simulink model "buck_discrete_pi_voltage_loop"  (R2024b)
settings: Solver=ode4  StartTime=0.0  StopTime=0.012  FixedStep=2.5e-7  RelTol=1e-3
undefined symbols (not defined in the file): DiscIntNeverNeededParam
settings Model: Creator=ww  LastModifiedBy=ww

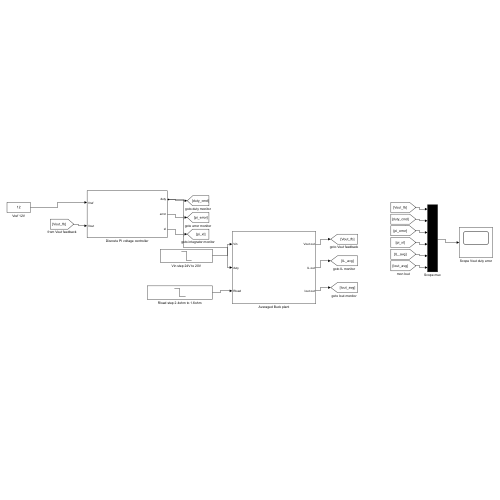
[thumbnail: Simulink's stored preview of the top-level diagram]
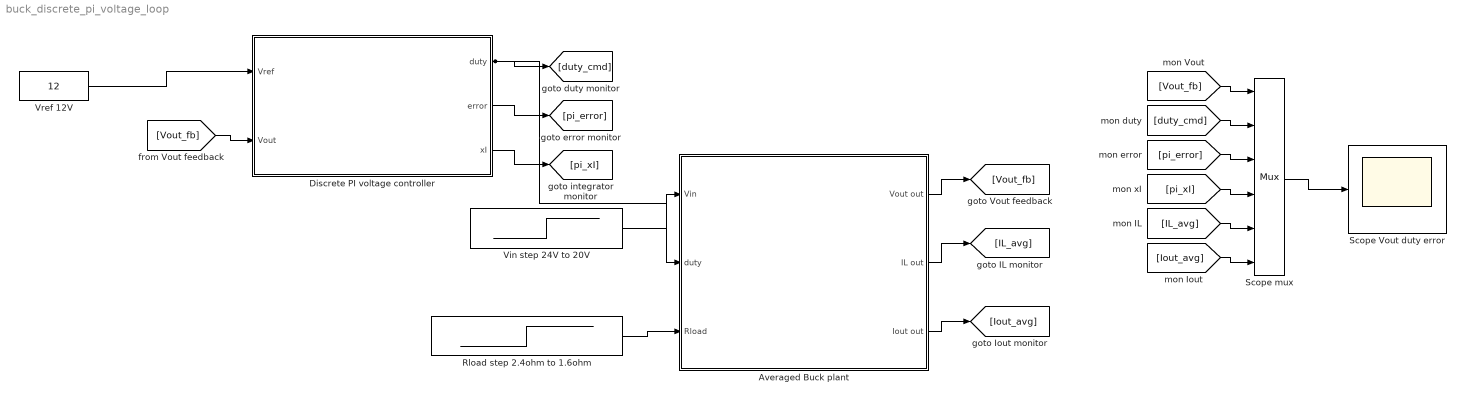
== system buck_discrete_pi_voltage_loop ==
  Averaged Buck plant : Subsystem
  Discrete PI voltage controller : Subsystem
  Rload step 2.4ohm to 1.6ohm : Step  Time=0.007  Before=2.4  After=1.6  SampleTime=0
  Scope Vout duty error : Scope
  Scope mux : Mux  Inputs=6
  Vin step 24V to 20V : Step  Time=0.003  Before=24  After=20  SampleTime=0
  Vref 12V : Constant  Value=12
  wires:
  [Vout_fb] -> Scope mux/1
  [duty_cmd] -> Scope mux/2
  [pi_error] -> Scope mux/3
  [pi_xI] -> Scope mux/4
  [IL_avg] -> Scope mux/5
  [Iout_avg] -> Scope mux/6
  Vref 12V/1 -> Discrete PI voltage controller/1(Vref)
  [Vout_fb] -> Discrete PI voltage controller/2(Vout)
  Discrete PI voltage controller/1(duty) -> Averaged Buck plant/2(duty), [duty_cmd]
  Vin step 24V to 20V/1 -> Averaged Buck plant/1(Vin)
  Rload step 2.4ohm to 1.6ohm/1 -> Averaged Buck plant/3(Rload)
  Discrete PI voltage controller/2(error) -> [pi_error]
  Discrete PI voltage controller/3(xI) -> [pi_xI]
  Averaged Buck plant/1(Vout out) -> [Vout_fb]
  Averaged Buck plant/2(IL out) -> [IL_avg]
  Averaged Buck plant/3(Iout out) -> [Iout_avg]
  Scope mux/1 -> Scope Vout duty error/1

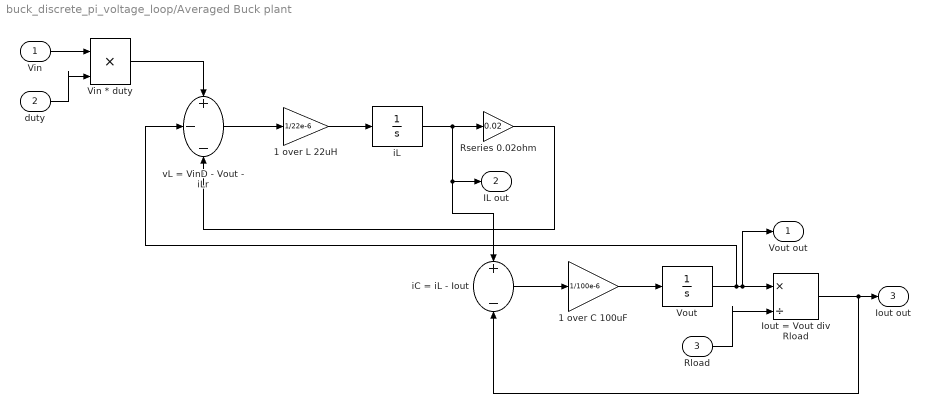
== system buck_discrete_pi_voltage_loop/Averaged Buck plant ==
  Vin : Inport
  duty : Inport  Port=2
  Rload : Inport  Port=3
  1 over C 100uF : Gain  Gain=1/100e-6
  1 over L 22uH : Gain  Gain=1/22e-6
  Iout = Vout div Rload : Product  Inputs=*/
  Rseries 0.02ohm : Gain  Gain=0.02
  Vin * duty : Product  Inputs=**
  Vout : Integrator  InitialCondition=12
  iC = iL - Iout : Sum  Inputs=+-
  iL : Integrator  InitialCondition=5
  vL = VinD - Vout - iLr : Sum  Inputs=+--
  Vout out : Outport
  IL out : Outport  Port=2
  Iout out : Outport  Port=3
  wires:
  duty/1 -> Vin * duty/2
  Vin/1 -> Vin * duty/1
  Vin * duty/1 -> vL = VinD - Vout - iLr/1
  vL = VinD - Vout - iLr/1 -> 1 over L 22uH/1
  1 over L 22uH/1 -> iL/1
  iL/1 -> iC = iL - Iout/1, IL out/1, Rseries 0.02ohm/1
  Iout = Vout div Rload/1 -> iC = iL - Iout/2, Iout out/1
  Rseries 0.02ohm/1 -> vL = VinD - Vout - iLr/3
  iC = iL - Iout/1 -> 1 over C 100uF/1
  1 over C 100uF/1 -> Vout/1
  Vout/1 -> Vout out/1, Iout = Vout div Rload/1, vL = VinD - Vout - iLr/2
  Rload/1 -> Iout = Vout div Rload/2

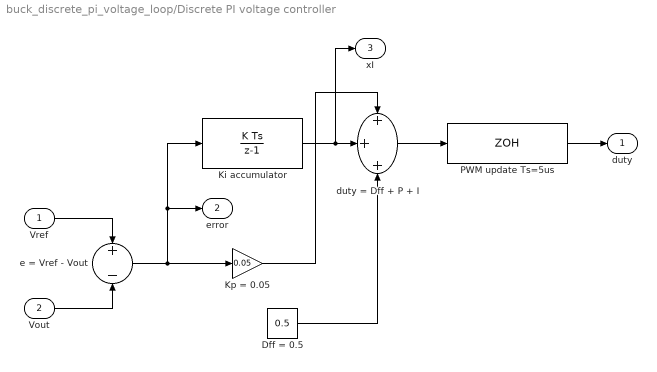
== system buck_discrete_pi_voltage_loop/Discrete PI voltage controller ==
  Vref : Inport
  Vout : Inport  Port=2
  Dff = 0.5 : Constant  Value=0.5
  Ki accumulator : DiscreteIntegrator  gainval=200  InitialCondition=0.0041667  SampleTime=5e-6  ICPrevOutput=DiscIntNeverNeededParam  ICPrevScaledInput=DiscIntNeverNeededParam
  Kp = 0.05 : Gain  Gain=0.05
  PWM update Ts=5us : ZeroOrderHold  SampleTime=5e-6
  duty = Dff + P + I : Sum  Inputs=+++
  e = Vref - Vout : Sum  Inputs=+-
  duty : Outport
  error : Outport  Port=2
  xI : Outport  Port=3
  wires:
  Vref/1 -> e = Vref - Vout/1
  Kp = 0.05/1 -> duty = Dff + P + I/1
  Ki accumulator/1 -> duty = Dff + P + I/2, xI/1
  Vout/1 -> e = Vref - Vout/2
  e = Vref - Vout/1 -> Ki accumulator/1, error/1, Kp = 0.05/1
  PWM update Ts=5us/1 -> duty/1
  duty = Dff + P + I/1 -> PWM update Ts=5us/1
  Dff = 0.5/1 -> duty = Dff + P + I/3
